simulink model "LQR_dlx_control"  (R2022b)
settings: Solver=VariableStepAuto  StartTime=0.0  StopTime=50  RelTol=1e-3
undefined symbols (not defined in the file): cx
libraries: Solver_SF x1, simulink x1
settings Model: Creator=admin  LastModifiedBy=admin

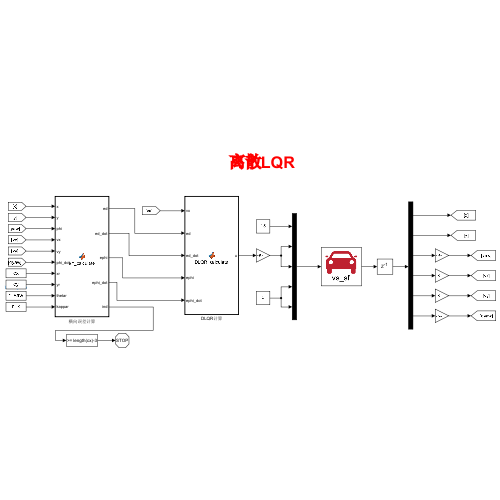
[thumbnail: Simulink's stored preview of the top-level diagram]
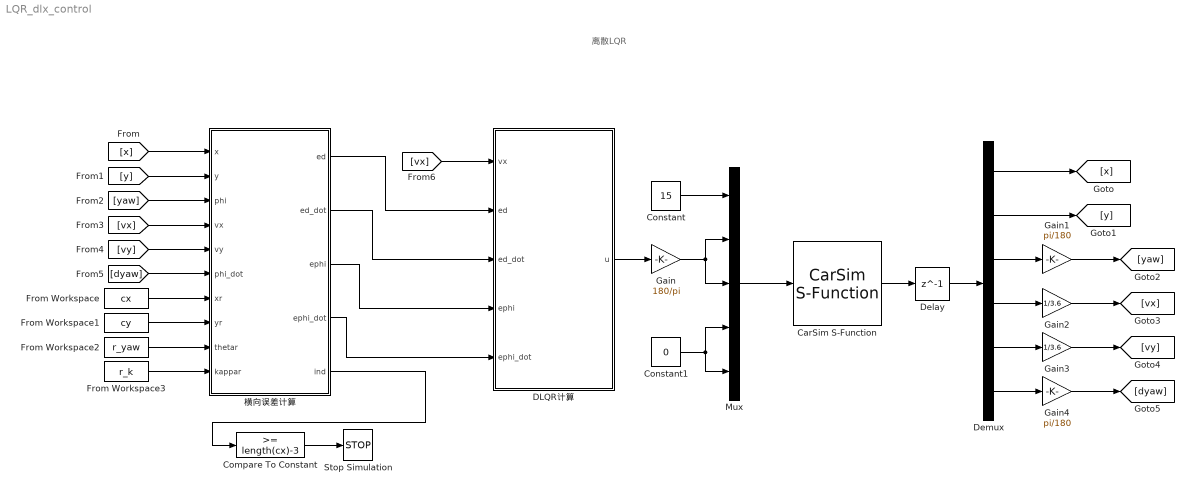
== system LQR_dlx_control ==
  note: 离散LQR
  CarSim S-Function : Solver_SF/CarSim S-Function  Priority=1  SIMFILE=simfile.sim  Run_RTs=off  vs_state_ind=Run  StopMode_ind=Vehicle Model
  Compare To Constant : simulink/Logic and Bit Operations/Compare To Constant  relop=>=  const=length(cx)-3  OutDataTypeStr=boolean
  Constant : Constant  Value=15
  Constant1 : Constant  Value=0
  DLQR计算 : MATLAB Function  TreatAsAtomicUnit=on
  Delay : Delay  DelayLength=1
  Demux : Demux  Outputs=6
  From Workspace : FromWorkspace  VariableName=cx
  From Workspace1 : FromWorkspace  VariableName=cy
  From Workspace2 : FromWorkspace  VariableName=r_yaw
  From Workspace3 : FromWorkspace  VariableName=r_k
  Gain : Gain  Gain=180/pi
  Gain1 : Gain  Gain=pi/180
  Gain2 : Gain  Gain=1/3.6
  Gain3 : Gain  Gain=1/3.6
  Gain4 : Gain  Gain=pi/180
  Mux : Mux  Inputs=5
  Stop Simulation : Stop
  横向误差计算 : MATLAB Function  TreatAsAtomicUnit=on
  wires:
  Constant/1 -> Mux/1
  Gain/1 -> Mux/3, Mux/2
  Constant1/1 -> Mux/5, Mux/4
  Mux/1 -> CarSim S-Function/1
  CarSim S-Function/1 -> Delay/1
  Delay/1 -> Demux/1
  Demux/1 -> [x]
  Demux/2 -> [y]
  Demux/3 -> Gain1/1
  Gain1/1 -> [yaw]
  Demux/4 -> Gain2/1
  Gain2/1 -> [vx]
  Demux/5 -> Gain3/1
  Gain3/1 -> [vy]
  Demux/6 -> Gain4/1
  Gain4/1 -> [dyaw]
  DLQR计算/1(u) -> Gain/1
  [x] -> 横向误差计算/1(x)
  [y] -> 横向误差计算/2(y)
  [yaw] -> 横向误差计算/3(phi)
  [vx] -> 横向误差计算/4(vx)
  [vy] -> 横向误差计算/5(vy)
  [dyaw] -> 横向误差计算/6(phi_dot)
  From Workspace/1 -> 横向误差计算/7(xr)
  From Workspace1/1 -> 横向误差计算/8(yr)
  From Workspace2/1 -> 横向误差计算/9(thetar)
  From Workspace3/1 -> 横向误差计算/10(kappar)
  Compare To Constant/1 -> Stop Simulation/1
  横向误差计算/5(ind) -> Compare To Constant/1
  [vx] -> DLQR计算/1(vx)
  横向误差计算/1(ed) -> DLQR计算/2(ed)
  横向误差计算/2(ed_dot) -> DLQR计算/3(ed_dot)
  横向误差计算/3(ephi) -> DLQR计算/4(ephi)
  横向误差计算/4(ephi_dot) -> DLQR计算/5(ephi_dot)

== matlab function LQR_dlx_control/DLQR计算 ==
  data: vx input; u output; ed input; ed_dot input; ephi input; ephi_dot input
% 首先在参考轨迹上搜索离当前车辆位置最近的点
function u   = DLQR_calculate(vx,ed,ed_dot,ephi, ephi_dot)
    e_X=[ed;ed_dot;ephi; ephi_dot];
    
    % 车辆参数
    cf = -79127;
    cr = -79127;
    m = 1235.9;
    Iz=1343.1;
    lf=1.3;
    lr=2.6-1.3;
    % 离散化采样时
    T=0.05; 
    
    v=vx+0.05;    % 分母不能为0，故加上很小数
    % 离散化之前的状态空间方程的矩阵系数 A,B
     a1=[0,          1,                  0,                  0;
         0,    (cf+cr)/(m*v),       -(cf+cr)/m,     (lf*cf-lr*cr)/(m*v);
         0,          0,                 0,                   1;
         0,(lf*cf-lr*cr)/(Iz*v),-(lf*cf-lr*cr)/Iz,(lf^2*cf+lr^2*cr)/(Iz*v)];
    
     b1=[   0;
          -cf/m;
            0;
        -lf*cf/Iz];
    % 离散化之后的状态空间方程的矩阵系数 A,B
     A = (eye(4)-a1*T/2)\(eye(4)+a1*T/2);  %中点欧拉法离散化
     B = T*b1;                             %向前欧拉法离散化
    
    % 由状态方程矩阵系数，计算K
        Q=1 *[30,0,0,0;
            0,5,0,0;
            0,0,5,0
            0,0,0,1];
        R=2;
    
    % 终止条件定义
    iter_max = 500;         %最大迭代次数
    epsilon = 0.01;         %容忍的最大误差
    
    % 求解反馈增益 K
    P_old = Q;
    for i = 1:iter_max
        P_new = A' * P_old * A - (A' * P_old * B) / (R + B' * P_old * B) *( B' * P_old * A) +Q;
        if abs(P_new - P_old) <= epsilon
            break
        else
            P_old = P_new; 
        end
    end
    
    P = P_new;
    K = (B' * P * B + R) \ (B' * P * A);  % 2行3列
    
    % 获得速度误差量、前轮转角误差量两个控制量
    u = -K * e_X;  % 2行1列

end

== matlab function LQR_dlx_control/横向误差计算 ==
  data: x input; ed output; y input; phi input; vx input; vy input; phi_dot input; xr input; yr input; thetar input; kappar input; ed_dot output; ephi output; ephi_dot output; ind output
function [ed,ed_dot,ephi,ephi_dot,ind] = err_calculate(x,y,phi, vx,vy,phi_dot,xr,yr,thetar,kappar)
    %寻找匹配点
    n=length(xr);
    d_min=(x-xr(1))^2+(y-yr(1))^2;
    min=1;
    for i=1:n
        d=(x-xr(i))^2+(y-yr(i))^2;
        if d<d_min
            d_min=d;
            min=i;
        end
    end
    ind=min;

    %计算状态方程中的状态向量
    tor=[cos(thetar(ind));sin(thetar(ind))];
    nor=[-sin(thetar(ind));cos(thetar(ind))];

    d_err=[x-xr(ind);y-yr(ind)]; 

    ed=nor'*d_err;                  %求取状态向量中的第一个 ed
    
    projection_point_thetar=thetar(ind); %百度apollo

    ed_dot=vy*cos(phi-projection_point_thetar)+vx*sin(phi-projection_point_thetar);%求取状态向量中的第二个 ed的导数

    ephi=sin(phi-projection_point_thetar);    %求取状态向量中的第三个 efai

    s_dot=vx*cos(phi-projection_point_thetar)-vy*sin(phi-projection_point_thetar);
    s_dot=s_dot/(1-kappar(ind)*ed);
    
    ephi_dot=phi_dot-kappar(ind)*s_dot;%求取状态向量中的第四个 efai 的倒数
end
